simulink model "METI_CVT_Thermal_ver01_2015a"  (R2015a)
settings: Solver=ode8  SolverMode=SingleTasking  StartTime=0  StopTime=1204  FixedStep=sampling_time  RelTol=1e-3
PreLoadFcn:
  | init_setting;
values from neighbouring files (symbols this model uses):
  degC2K = 273.15    [METI_TRAMI_Thermal_ver01_Jmaab_PreLoad.m]    (also in init_setting_METI.m)
  K2degC = -273.15    [METI_TRAMI_Thermal_ver01_Jmaab_PreLoad.m]    (also in init_setting_METI.m)
  sampling_time = 0.0025    [METI_TRAMI_Thermal_ver01_Jmaab_PreLoad.m]
undefined symbols (not defined in the file or in its folder): ALT_CNT_ALT_OFF_RPM_HYS_rpm, ALT_CNT_ALT_ON_RPM_HYS_rpm, ALT_CNT_Alter_V_BASE_V, ALT_CNT_Alter_V_Kaisei_V, ALT_CNT_flag_disable_kaisei, ALT_CNT_V_Battely_Kudo_V, ALT_PNT_ALT_GDCurrent_A, ALT_PNT_ALT_GDVolt_V, ALT_PNT_Alter_limit_Current_V_table, ALT_PNT_Alter_limit_Current_V_table_x_rpm, ALT_PNT_Alter_trq_Nm_map, ALT_PNT_Alter_trq_Nm_map_x_rpm, ALT_PNT_Alter_trq_Nm_map_y_Current_A, ALT_PNT_Alter_trq_Nm_map_z_Volt_tgt_V, ALT_PNT_eta_pulley_alt, ALT_PNT_Gain_Alt_v_del, ALT_PNT_ratio_pulley_alt, ALT_PNT_Tau_Alternator_V_tgt_s, ALT_PNT_trq_alter_output_LL_Nm, BK_PNT_Pow_UL, BK_PNT_Tau_brake, Brk_LL, Brk_PGain, Brk_UL, BT_PNT_Lo_Capa_lo_batt_F, BT_PNT_Lo_ocv_SOC_lo_batt_OCV_V_table, BT_PNT_Lo_ocv_SOC_lo_batt_OCV_V_table_x_SOC, BT_PNT_Lo_R_lo_batt_ohm, BT_PNT_Lo_SOC_MAX_lo_batt, BT_PNT_Lo_SOC_MIN_lo_batt, BT_PNT_Lo_SOC_START_lo_batt, DF_PNT_DF_gear, DF_PNT_DFBlock2DFAir_Heat_Resi_KpW, DF_PNT_DFBlock_Heat_Capa_JpK, DF_PNT_DFBlock_Temp_ini_degC, DF_PNT_DFOil2DFBlock_Heat_Resi_KpW, DF_PNT_DFOil_Heat_Capa_JpK, DF_PNT_DFOil_Temp_ini_degC, DF_PNT_Driveshaft_damper, DF_PNT_Driveshaft_delta_radps_LL, DF_PNT_Driveshaft_delta_radps_UL, DF_PNT_Driveshaft_spring, DF_PNT_eta_DF, DF_PNT_Outtemp_degC, DF_PNT_TMBlock2DFBlock_Heat_Resi_KpW, Driver_Brake_Const1, Driver_Brake_Const3, Driver_Brake_Switch_Const2, Driver_Brk_sh, drivmode_ACC, drivmode_CONST, drivmode_GensokuKaisei, drivmode_GensokuRikko, drivmode_STOP, EL_PNT_R_bodyelec_lo_ohm, ENG_CNT_acc_idlestop, ENG_CNT_Accel_LL, ENG_CNT_Accel_UL, ENG_CNT_brak_idlestop, ENG_CNT_flag_idle_stop_exe ... (+133)
undefined symbols (not defined in the file): ACC_D_Gain, ACC_I_Gain, ACC_P_Gain
libraries: METI_Lib_vehicle_model x32, simulink x7, AZAPA_Lib_vehicle_model x1
(part 1 of 3)
settings Model: CovSFcnEnable=off  Creator=nishimura  LastModifiedBy=AZ064
settings OptimizationCC: BlockReduction=off  BooleanDataType=off  EfficientMapNaN2IntZero=off
settings DebuggingCC: SaveWithParameterizedLinksMsg=none  UnderspecifiedInitializationDetection=Classic  MergeDetectMultiDrivingBlocksExec=none  SignalResolutionControl=TryResolveAllWithWarning  StrictBusMsg=ErrorOnBusTreatedAsVector
settings HardwareCC: TargetLongLongMode=on  TargetIntDivRoundTo=Zero  TargetEndianess=LittleEndian  TargetHWDeviceType=MATLAB Host  ProdEqTarget=off
settings CodeAppCC: MaxIdLength=128
settings GRTTargetCC: CombineOutputUpdateFcns=off  GRTInterface=on

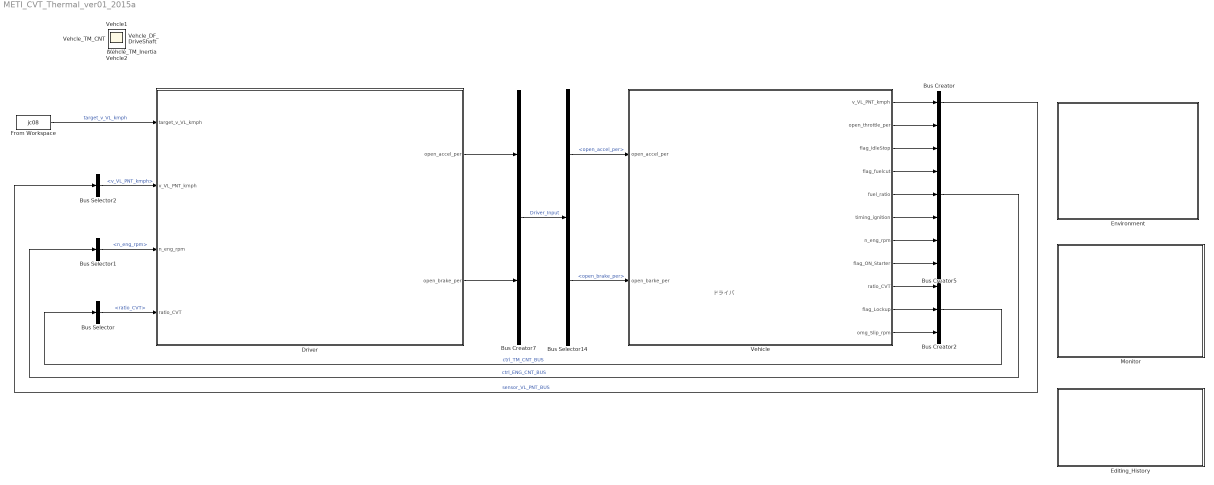
== system METI_CVT_Thermal_ver01_2015a ==
  note: ドライバ
  Bus Creator : BusCreator  Inputs=1
  Bus Creator2 : BusCreator  Inputs=3
  Bus Creator5 : BusCreator  Inputs=7
  Bus Creator7 : BusCreator  Inputs=2
  Bus Selector : BusSelector  OutputSignals=ratio_CVT
  Bus Selector1 : BusSelector  OutputSignals=n_eng_rpm
  Bus Selector14 : BusSelector  OutputSignals=open_accel_per,open_brake_per
  Bus Selector2 : BusSelector  OutputSignals=v_VL_PNT_kmph
  Driver : Subsystem
      mask Display: image(imread('picture\ドライバ.png'))
  Editing_History : Subsystem
  Environment : Subsystem
      mask Display: image(imread('picture\外部環境.png'))
  From Workspace : FromWorkspace  VariableName=jc08  SampleTime=0  OutputAfterFinalValue=Holding final value
  Monitor : Subsystem
  Vehicle : Subsystem
      mask Display: image(imread('picture\電気負荷.png'))
  Driver1 : Scope
      settings: YMin=-12.5  YMax=112.5  SaveName=ScopeData2
  Vehcle1 : Scope
      settings: YMin=-10  YMax=10  SaveName=ScopeData8
  Vehcle2 : Scope
      settings: YMin=-19.56201  YMax=196.87604
  Vehcle_DF_DriveShaft : Scope
      settings: YMin=-11.28415  YMax=101.55731  SaveName=ScopeData6
  Vehcle_TM_CNT : Scope
      settings: YMin=-0.125  YMax=1.125  SaveName=ScopeData8
  Vehcle_TM_Inertia : Scope
      settings: YMin=-138.01223  YMax=25.56889  SaveName=ScopeData7
  wires:
  From Workspace/1 -> Driver/1(target_v_VL_kmph)  "target_v_VL_kmph"
  Bus Creator7/1 -> Bus Selector14/1  "Driver_Input"
  Bus Creator/1 -> Bus Selector2/1  "sensor_VL_PNT_BUS"
  Bus Creator2/1 -> Bus Selector/1  "ctrl_TM_CNT_BUS"
  Bus Creator5/1 -> Bus Selector1/1  "ctrl_ENG_CNT_BUS"
  Vehicle/1(v_VL_PNT_kmph) -> Bus Creator/1
  Vehicle/2(open_throttle_per) -> Bus Creator5/1
  Vehicle/3(flag_IdleStop) -> Bus Creator5/2
  Vehicle/4(flag_fuelcut) -> Bus Creator5/3
  Vehicle/5(fuel_ratio) -> Bus Creator5/4
  Vehicle/6(timing_ignition) -> Bus Creator5/5
  Vehicle/7(n_eng_rpm) -> Bus Creator5/6
  Vehicle/8(flag_ON_Starter) -> Bus Creator5/7
  Vehicle/10(flag_Lockup) -> Bus Creator2/2
  Vehicle/9(ratio_CVT) -> Bus Creator2/1
  Vehicle/11(omg_Slip_rpm) -> Bus Creator2/3
  Bus Selector14/1 -> Vehicle/1(open_accel_per)  "<open_accel_per>"
  Bus Selector14/2 -> Vehicle/2(open_barke_per)  "<open_brake_per>"
  Driver/1(open_accel_per) -> Bus Creator7/1
  Driver/2(open_brake_per) -> Bus Creator7/2
  Bus Selector/1 -> Driver/4(ratio_CVT)  "<ratio_CVT>"
  Bus Selector1/1 -> Driver/3(n_eng_rpm)  "<n_eng_rpm>"
  Bus Selector2/1 -> Driver/2(v_VL_PNT_kmph)  "<v_VL_PNT_kmph>"

== system METI_CVT_Thermal_ver01_2015a/Driver ==
  note: ドライバモデルのへたくそ対応
  note: 全体としてパワーを算出しておいて、
      | さらにパワーと速度のF/Bを切り替えれるようにしておく
  target_v_VL_kmph : Inport
  v_VL_PNT_kmph : Inport  Port=2
  n_eng_rpm : Inport  Port=3
  ratio_CVT : Inport  Port=4
  Caliculate_Driving_State : Subsystem
  Caliculate_Opeining_Accel : Subsystem
  Caliculate_Opening_Brake : Subsystem
  Memory2 : Memory  InheritSampleTime=on
  Memory3 : Memory
  Memory4 : Memory
  open_accel_per : Outport
  open_brake_per : Outport  Port=2
  tag scope: tScope_accel=global, tScope_brake=global
  wires:
  target_v_VL_kmph/1 -> Caliculate_Opeining_Accel/2(target_v_VL_kmph), Caliculate_Opening_Brake/2(target_v_VL_kmph), Caliculate_Driving_State/2(target_v_VL_kmph)
  Memory3/1 -> Caliculate_Opeining_Accel/3(pre_n_eng_rpm)  "pre_n_eng_rpm"
  ratio_CVT/1 -> Memory4/1
  Memory4/1 -> Caliculate_Opeining_Accel/4(pre_ratio_CVT)  "pre_ratio_CVT"
  n_eng_rpm/1 -> Memory3/1
  Memory2/1 -> Caliculate_Opening_Brake/1(v_VL_PNT_kmph), Caliculate_Opeining_Accel/1(v_VL_PNT_kmph)
  Caliculate_Opeining_Accel/1(open_accel_per) -> Caliculate_Opening_Brake/3(open_accel_per), open_accel_per/1, [tScope_accel]
  Caliculate_Opening_Brake/1(open_brake_per) -> Caliculate_Driving_State/1(open_brake_per), open_brake_per/1, [tScope_brake]
  v_VL_PNT_kmph/1 -> Memory2/1

== system METI_CVT_Thermal_ver01_2015a/Editing_History ==
  note: 編集履歴
      |
      | 2019/3/29　初版
      |
      | 2019/7/3　ver.2
      | ・ENG_CNT内部と出力の結線名を修正
      | ・DFとPTTH間の熱のI/Fを追加修正
      | ・PTTH_PNT/RDTH_PNTの絵が同梱されていなかったため追加

== system METI_CVT_Thermal_ver01_2015a/Environment ==
  note: 登坂。風、温度、湿度・・・
  Clock : Clock
  To Workspace : ToWorkspace  VariableName=simtime  SampleTime=-1
      settings: Decimation=num_tws_mabiki
  wires:
  Clock/1 -> To Workspace/1

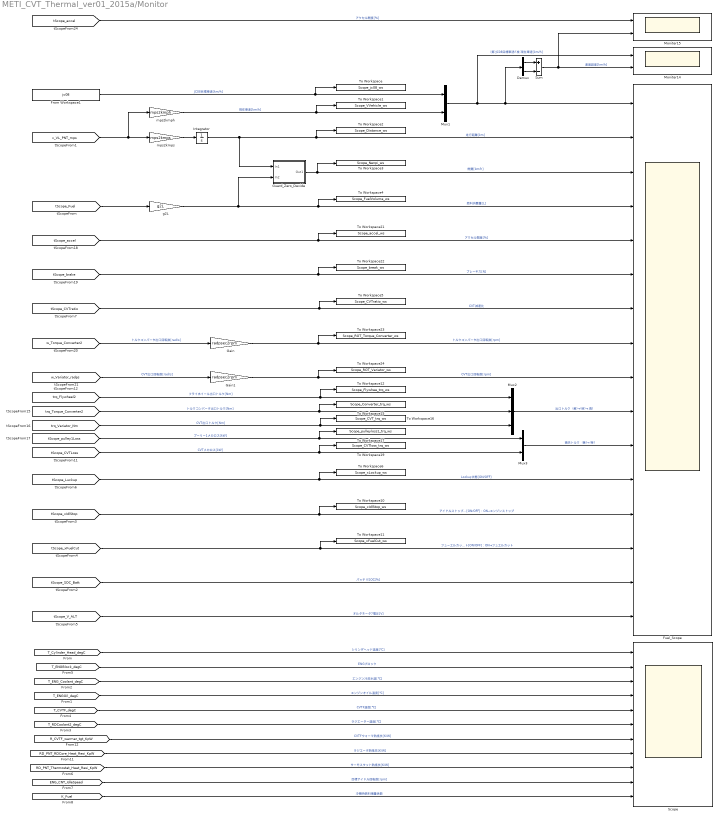
== system METI_CVT_Thermal_ver01_2015a/Monitor ==
  Demux : Demux  Outputs=2
  From Workspace1 : FromWorkspace  VariableName=jc08  SampleTime=0  OutputAfterFinalValue=Holding final value
  Fuel_Scope : Scope  NumInputPorts=16
      settings: YMin=0~0~0~0~0~0~0.25~0~0~-300~-500~0~0~0~99.6~9  YMax=75~5~20~0.3~20~100~2.5~4000~5000~300~3500~1~1~1~100.3~15
  Gain : Gain  Gain=radpsec2rpm
  Gain1 : Gain  Gain=radpsec2rpm
  Guard_Zero_Devide : Subsystem
  Integrator : Integrator
  Moniter14 : Scope  NumInputPorts=2
      settings: YMin=-10.20589~-3.34691  YMax=91.85305~1.30656
  Moniter15 : Scope  NumInputPorts=2
      settings: YMin=-1.14178~-3.31361  YMax=10.27601~1.05767
  Mux1 : Mux  Inputs=2
  Mux2 : Mux  Inputs=3
  Mux3 : Mux  Inputs=2
  Scope : Scope  NumInputPorts=11
      settings: YMin=0~25~25~25~25~25~-5~-5~-5~-5~-5  YMax=1050~125~100~100~100~100~5~5~5~5~5  SaveName=ScopeData3  Decimation=10
  Sum : Sum  Inputs=+-
  To Workspace : ToWorkspace  VariableName=Scope_jc08_ws  SaveFormat=Structure With Time  SampleTime=-1
      settings: Decimation=num_tws_mabiki
  To Workspace1 : ToWorkspace  VariableName=Scope_VVehicle_ws  SaveFormat=Structure With Time  SampleTime=-1
      settings: Decimation=num_tws_mabiki
  To Workspace10 : ToWorkspace  VariableName=Scope_xIdlStop_ws  SaveFormat=Structure With Time  SampleTime=-1
      settings: Decimation=num_tws_mabiki
  To Workspace11 : ToWorkspace  VariableName=Scope_xFuelCut_ws  SaveFormat=Structure With Time  SampleTime=-1
      settings: Decimation=num_tws_mabiki
  To Workspace12 : ToWorkspace  VariableName=Scope_Flywhee_trq_ws  SaveFormat=Structure With Time  SampleTime=-1
      settings: Decimation=num_tws_mabiki
  To Workspace15 : ToWorkspace  VariableName=Scope_Converter_trq_ws  SaveFormat=Structure With Time  SampleTime=-1
      settings: Decimation=num_tws_mabiki
  To Workspace16 : ToWorkspace  VariableName=Scope_CVT_trq_ws  SaveFormat=Structure With Time  SampleTime=-1
      settings: Decimation=num_tws_mabiki
  To Workspace17 : ToWorkspace  VariableName=Scope_pulleyloss1_trq_ws  SaveFormat=Structure With Time  SampleTime=-1
      settings: Decimation=num_tws_mabiki
  To Workspace19 : ToWorkspace  VariableName=Scope_CVTloss_trq_ws  SaveFormat=Structure With Time  SampleTime=-1
      settings: Decimation=num_tws_mabiki
  To Workspace2 : ToWorkspace  VariableName=Scope_Distance_ws  SaveFormat=Structure With Time  SampleTime=-1
      settings: Decimation=num_tws_mabiki
  To Workspace21 : ToWorkspace  VariableName=Scope_accel_ws  SaveFormat=Structure With Time  SampleTime=-1
      settings: Decimation=num_tws_mabiki
  To Workspace22 : ToWorkspace  VariableName=Scope_break_ws  SaveFormat=Structure With Time  SampleTime=-1
      settings: Decimation=num_tws_mabiki
  To Workspace23 : ToWorkspace  VariableName=Scope_ROT_Torque_Converter_ws  SaveFormat=Structure With Time  SampleTime=-1
      settings: Decimation=num_tws_mabiki
  To Workspace24 : ToWorkspace  VariableName=Scope_ROT_Variator_ws  SaveFormat=Structure With Time  SampleTime=-1
      settings: Decimation=num_tws_mabiki
  To Workspace3 : ToWorkspace  VariableName=Scope_Nenpi_ws  SaveFormat=Structure With Time  SampleTime=-1
      settings: Decimation=num_tws_mabiki
  To Workspace4 : ToWorkspace  VariableName=Scope_FuelVolume_ws  SaveFormat=Structure With Time  SampleTime=-1
      settings: Decimation=num_tws_mabiki
  To Workspace5 : ToWorkspace  VariableName=Scope_CVTratio_ws  SaveFormat=Structure With Time  SampleTime=-1
      settings: Decimation=num_tws_mabiki
  To Workspace6 : ToWorkspace  VariableName=Scope_xLockup_ws  SaveFormat=Structure With Time  SampleTime=-1
      settings: Decimation=num_tws_mabiki
  g2L : Gain  Gain=g2L
  mps2kmph : Gain  Gain=mps2kmph
  mps2kmps : Gain  Gain=mps2kmps
  wires:
  [tScope_xIdlStop] -> To Workspace10/1, Fuel_Scope/13  "アイドルストップ[ON/OFF] : ON→エンジンストップ"
  [tScope_xFuelCut] -> To Workspace11/1, Fuel_Scope/14  "フューエルカット[ON/OFF] : ON→フュエルカット"
  [v_VL_PNT_mps] -> mps2kmph/1, mps2kmps/1
  mps2kmps/1 -> Integrator/1
  [tScope_Fuel] -> g2L/1
  Integrator/1 -> Guard_Zero_Devide/1(In1), To Workspace2/1, Fuel_Scope/2  "走行距離[km]"
  g2L/1 -> To Workspace4/1, Fuel_Scope/4, Guard_Zero_Devide/2(In2)  "燃料消費量[L]"
  [tScope_Luckup] -> To Workspace6/1, Fuel_Scope/12  "Lockup状態[ON/OFF]"
  [tScope_CVTratio] -> To Workspace5/1, Fuel_Scope/7  "CVT減速比"
  From Workspace1/1 -> To Workspace/1, Mux1/1  "JC08目標車速[km/h]"
  mps2kmph/1 -> To Workspace1/1, Mux1/2  "現在車速[km/h]"
  Mux1/1 -> Moniter14/1, Demux/1, Fuel_Scope/1  "(黄)JC08目標車速/(桃)現在車速[km/h]"
  [tScope_CVTLoss] -> To Workspace19/1, Mux3/2  "CVTメカロス[kW]"
  [trq_Flywheel2] -> To Workspace12/1, Mux2/1  "フライホイール出口トルク[Nm]"
  [trq_Torque_Converter2] -> To Workspace15/1, Mux2/2  "トルクコンバータ出口トルク[Nm]"
  [trq_Variator_Nm] -> To Workspace16/1, Mux2/3  "CVT出口トルク[Nm]"
  [tScope_pulley1Loss] -> To Workspace17/1, Mux3/1  "プーリー1メカロス[kW]"
  Mux2/1 -> Fuel_Scope/10  "出口トルク  (黄)→(桃)→(青)"
  Mux3/1 -> Fuel_Scope/11  "損失トルク  (黄)→(桃)"
  [tScope_accel] -> To Workspace21/1, Fuel_Scope/5  "アクセル開度[%]"
  [tScope_brake] -> To Workspace22/1, Fuel_Scope/6  "ブレーキ力[N]"
  Gain/1 -> Fuel_Scope/8, To Workspace23/1  "トルクコンバータ出口回転数[rpm]"
  [w_Variator_radps] -> Gain1/1  "CVT出口回転数[rad/s]"
  Demux/1 -> Sum/1
  Demux/2 -> Sum/2
  Sum/1 -> Moniter14/2, Moniter15/2  "速度誤差[km/h]"
  [tScope_accel] -> Moniter15/1  "アクセル開度[%]"
  [tScope_V_ALT] -> Fuel_Scope/16  "オルタネータ7電圧[V]"
  [tScope_SOC_Batt] -> Fuel_Scope/15  "バッテリSOC[%]"
  Guard_Zero_Devide/1(Out1) -> To Workspace3/1, Fuel_Scope/3  "燃費[km/h]"
  [T_CVTF_degC] -> Scope/5  "CVTF温度[℃]"
  [T_RDCoolant2_degC] -> Scope/6  "ラジエーター温度[℃]"
  [T_ENG_Coolant_degC] -> Scope/3  "エンジン冷却水温[℃]"
  [T_ENGOil_degC] -> Scope/4  "エンジンオイル温度[℃]"
  [T_Cylinder_Head_degC] -> Scope/1  "シリンダヘッド温度[℃]"
  [T_ENGBlock_degC] -> Scope/2  "ENGブロック"
  [w_Torque_Converter2] -> Gain/1  "トルクコンバータ出口回転数[rad/s]"
  Gain1/1 -> To Workspace24/1, Fuel_Scope/9  "CVT出口回転数[rpm]"
  [R_CVTF_warmer_tgt_KpW] -> Scope/7  "CVTFウォーマ熱抵抗[K/W]"
  [RD_PNT_RDCore_Heat_Resi_KpW] -> Scope/8  "ラジエータ熱抵抗[K/W]"
  [RD_PNT_Thermostat_Heat_Resi_KpW] -> Scope/9  "サーモスタット熱抵抗[K/W]"
  [ENG_CNT_IdleSpeed] -> Scope/10  "目標アイドル回転数[rpm]"
  [K_Fuel] -> Scope/11  "冷機時燃料増量係数"

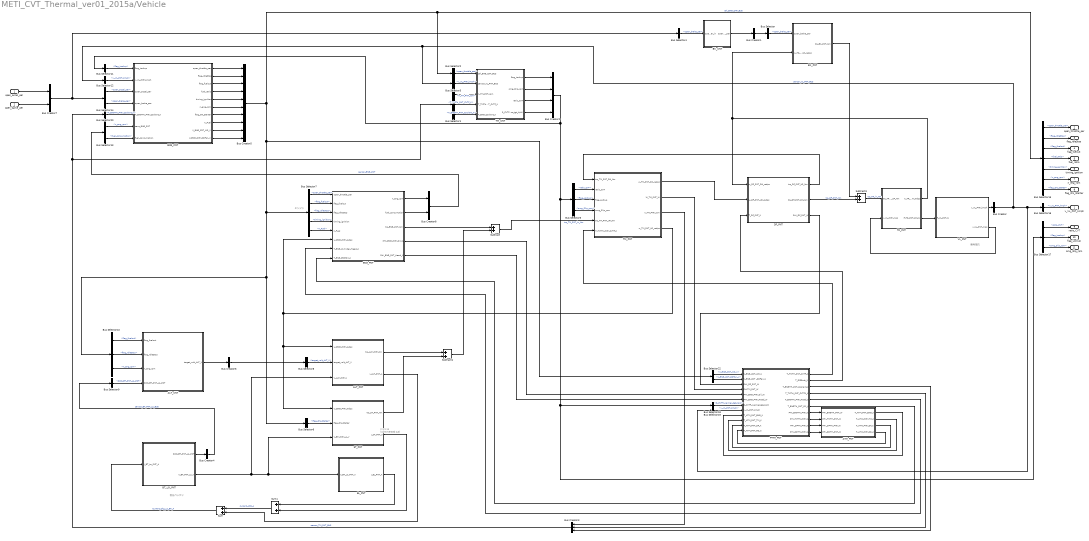
== system METI_CVT_Thermal_ver01_2015a/Vehicle ==
  note: エンジン
  note: 車両抵抗
  note: 低圧バッテリ
  open_accel_per : Inport
  open_barke_per : Inport  Port=2
  ALT_CNT : Subsystem
      mask Display: image(imread('picture\ECU.png'))
  ALT_PNT : Subsystem
      mask Display: image(imread('picture\image\オルタネータ02.jpg'))
  ATM_PNT : Subsystem
  BK_CNT : Subsystem
      mask Display: image(imread('picture\ECU.png'))
  BK_PNT : Subsystem
      mask Display: image(imread('picture\ブレーキ02.png'))
  BT_LO_PNT : Subsystem
      mask Display: image(imread('picture\バッテリー.png'))
  Bus Creator{,1,4,6} (4 alike) : BusCreator  Inputs=1
  Bus Creator2 : BusCreator
  Bus Creator3 : BusCreator  Inputs=3
  Bus Creator5 : BusCreator  Inputs=10
  Bus Creator7 : BusCreator  Inputs=2
  Bus Creator8 : BusCreator  Inputs=2
  Bus Selector : BusSelector  OutputSignals=open_brake_per
  Bus Selector1 : BusSelector  OutputSignals=n_TM_PNT_rpm,T_TMTH_PNT_CVTF_K,T_ENGTH_PNT_Coolant_K
  Bus Selector10 : BusSelector  OutputSignals=flag_fuelcut,flag_IdleStop,n_eng_rpm
  Bus Selector11 : BusSelector  OutputSignals=flag_Lockup
  Bus Selector{3,12,16,19} (4 alike) : BusSelector  OutputSignals=v_VL_PNT_kmph
  Bus Selector13 : BusSelector  OutputSignals=n_eng_rpm,fuel_consumption
  Bus Selector14 : BusSelector  OutputSignals=open_accel_per,open_brake_per
  Bus Selector15 : BusSelector  OutputSignals=open_throttle_per,flag_IdleStop,flag_fuelcut,fuel_ratio,timing_ignition,n_eng_rpm,flag_ON_Starter
  Bus Selector17 : BusSelector  OutputSignals=ratio_CVT,flag_Lockup,omg_Slip_rpm
  Bus Selector18 : BusSelector  OutputSignals=R_CVTF_warmer_tgt_KpW
  Bus Selector2 : BusSelector  OutputSignals=open_throttle_per
  Bus Selector20 : BusSelector  OutputSignals=T_ENGTH_PNT_Coolant_K
  Bus Selector22 : BusSelector  OutputSignals=V_ENG_CNT_WP_V,V_ENG_CNT_RDFan_V
  Bus Selector4 : BusSelector  OutputSignals=open_brake_per
  Bus Selector5 : BusSelector  OutputSignals=ratio_CVT,flag_Lockup,omg_Slip_rpm
  Bus Selector6 : BusSelector  OutputSignals=flag_ON_Starter
  Bus Selector7 : BusSelector  OutputSignals=open_throttle_per,flag_fuelcut,flag_IdleStop,timing_ignition,K_Fuel
  Bus Selector8 : BusSelector  OutputSignals=target_volt_ALT_V
  Bus Selector9 : BusSelector  OutputSignals=SOC_BT_PNT_Lo_PCT
  DF_PNT : Subsystem
      mask Display: image(imread('picture\回転変換.png'))
  EL_PNT : Subsystem
      mask Display: image(imread('picture\電気負荷.png'))
  ENG_CNT : Subsystem
      mask Display: image(imread('picture\ECU.png'))
  ENG_PNT : Subsystem
      mask Display: image(imread('picture\image\エンジン03.jpg'))
  From15 : From  Commented=on  GotoTag=I_ST_PNT_A  TagVisibility=global
  PTTH_PNT : Subsystem
  ST_PNT : Subsystem
      mask Display: image(imread('picture\image\スターター02.jpg'))
  Subtract : Sum  Inputs=2
  Subtract1 : Sum  Inputs=2
  Subtract3 : Sum  Inputs=2
  Sum : Sum
  Sum1 : Sum
  TM_CNT : Subsystem
      mask Display: image(imread('picture\ECU.png'))
  TM_PNT : Subsystem
      mask Display: image(imread('picture\image\トランスミッション02.jpg'))
  TR_PNT : Subsystem
      mask Display: image(imread('picture\タイヤ01.png'))
  VL_PNT : Subsystem
      mask Display: image(imread('picture\車両抵抗.png'))
  v_VL_PNT_kmph : Outport
  open_throttle_per : Outport  Port=2
  flag_IdleStop : Outport  Port=3
  flag_fuelcut : Outport  Port=4
  fuel_ratio : Outport  Port=5
  timing_ignition : Outport  Port=6
  n_eng_rpm : Outport  Port=7
  flag_ON_Starter : Outport  Port=8
  ratio_CVT : Outport  Port=9
  flag_Lockup : Outport  Port=10
  omg_Slip_rpm : Outport  Port=11
  wires:
  Bus Creator7/1 -> Bus Selector4/1, Bus Selector14/1
  Sum/1 -> BT_LO_PNT/1(I_BT_Lo_PNT_A)  "Current_Chg_Lo_BT_A"
  EL_PNT/1(I_EL_PNT_A) -> Sum1/1
  ALT_PNT/2(I_ALT_PNT_A) -> Sum/2
  Bus Creator5/1 -> Bus Selector15/1, Bus Selector2/1, Bus Selector22/1, Bus Selector7/1, Bus Selector6/1, Bus Selector10/1  "ctrl_ENG_CNT_BUS"
  Bus Creator6/1 -> Bus Selector8/1
  ST_PNT/2(I_ST_PNT_A) -> Sum1/2
  BT_LO_PNT/2(V_BT_PNT_Lo_V) -> ALT_PNT/3(V_ALT_PNT_V), EL_PNT/1(V_BT_Lo_PNT_V), ST_PNT/3(V_BT_PNT_Lo_V)
  Subtract/1 -> TM_PNT/5(trq_TM_PNT_UP_Nm)  "trq_TM_PNT_in_Nm"
  Bus Creator3/1 -> Bus Selector20/1, Bus Selector1/1  "sensor_TM_PNT_BUS"
  ENG_PNT/3(trq_ENG_PNT_Nm) -> Subtract/1
  Bus Creator2/1 -> Bus Selector17/1, Bus Selector18/1, Bus Selector5/1, Bus Selector11/1
  Bus Creator/1 -> Bus Selector16/1, Bus Selector19/1, Bus Selector3/1, Bus Selector12/1  "sensor_VL_PNT_BUS"
  BK_PNT/1(trq_BK_PNT_Nm) -> Subtract3/1
  TR_PNT/2(F_TR_PNT_DN_N) -> VL_PNT/1(F_VL_PNT_N)
  Subtract3/1 -> TR_PNT/1(trq_TR_PNT_UP_Nm)  "trq_TR_in_Nm"
  VL_PNT/2(v_VL_PNT_mps) -> TR_PNT/2(v_VL_PNT_mps)
  VL_PNT/1(v_VL_PNT_kmph) -> Bus Creator/1
  Bus Creator1/1 -> Bus Selector/1
  BK_CNT/1(open_brake_per) -> Bus Creator1/1
  Bus Selector/1 -> BK_PNT/1(open_brake_per)  "<open_brake_per>"
  Bus Selector1/1 -> TM_CNT/3(n_TM_PNT_rpm)  "<n_TM_PNT_rpm>"
  Bus Selector2/1 -> TM_CNT/1(ctrl_ENG_CNT_BUS)  "<open_throttle_per>"
  Bus Selector3/1 -> TM_CNT/2(sensor_VL_PNT_BUS)  "<v_VL_PNT_kmph>"
  TM_CNT/1(flag_Lockup) -> Bus Creator2/1
  TM_CNT/2(omg_Slip_rpm) -> Bus Creator2/2
  TM_CNT/3(ratio_CVT) -> Bus Creator2/3
  Bus Selector4/1 -> BK_CNT/1(open_brake_per_in)  "<open_brake_per>"
  Bus Selector5/1 -> TM_PNT/2(ratio_CVT)  "<ratio_CVT>"
  Bus Selector5/2 -> TM_PNT/3(flag_Lockup)  "<flag_Lockup>"
  Bus Selector5/3 -> TM_PNT/4(omg_Slip_rpm)  "<omg_Slip_rpm>"
  TM_PNT/3(n_TM_PNT_rpm) -> Bus Creator3/1
  Bus Creator4/1 -> Bus Selector9/1  "sensor_BT_PNT_Lo_BUS"
  BT_LO_PNT/1(SOC_BT_PNT_Lo_PCT) -> Bus Creator4/1
  Bus Selector6/1 -> ST_PNT/2(flag_ON_Starter)  "<flag_ON_Starter>"
  Bus Selector7/1 -> ENG_PNT/1(open_throttle_per)  "<open_throttle_per>"
  Bus Selector7/2 -> ENG_PNT/2(flag_fuelcut)  "<flag_fuelcut>"
  Bus Selector7/3 -> ENG_PNT/3(flag_IdleStop)  "<flag_IdleStop>"
  Bus Selector7/4 -> ENG_PNT/4(timing_ignition)  "<timing_ignition>"
  ENG_CNT/1(open_throttle_per) -> Bus Creator5/1
  ENG_CNT/7(flag_ON_Starter) -> Bus Creator5/7
  ENG_CNT/6(n_eng_rpm) -> Bus Creator5/6
  ENG_CNT/5(timing_ignition) -> Bus Creator5/5
  ENG_CNT/4(fuel_ratio) -> Bus Creator5/4
  ENG_CNT/3(flag_fuelcut) -> Bus Creator5/3
  ENG_CNT/2(flag_IdleStop) -> Bus Creator5/2
  Bus Selector8/1 -> ALT_PNT/2(target_volt_ALT_V)  "<target_volt_ALT_V>"
  ALT_CNT/1(target_volt_ALT_V) -> Bus Creator6/1
  Bus Selector9/1 -> ALT_CNT/4(SOC_BT_PNT_Lo_PCT)  "<SOC_BT_PNT_Lo_PCT>"
  Bus Selector10/1 -> ALT_CNT/1(flag_fuelcut)  "<flag_fuelcut>"
  Bus Selector10/2 -> ALT_CNT/2(flag_IdleStop)  "<flag_IdleStop>"
  Bus Selector10/3 -> ALT_CNT/3(n_eng_rpm)  "<n_eng_rpm>"
  Bus Selector11/1 -> ENG_CNT/1(flag_Lockup)  "<flag_Lockup>"
  Bus Selector12/1 -> ENG_CNT/2(v_VL_PNT_kmph)  "<v_VL_PNT_kmph>"
  Bus Selector13/1 -> ENG_CNT/6(sens_ENG_PNT)  "<n_eng_rpm>"
  Bus Selector14/1 -> ENG_CNT/3(open_accel_per)  "<open_accel_per>"
  Bus Selector14/2 -> ENG_CNT/4(open_brake_per)  "<open_brake_per>"
  Bus Selector16/1 -> v_VL_PNT_kmph/1  "<v_VL_PNT_kmph>"
  Bus Selector15/1 -> open_throttle_per/1  "<open_throttle_per>"
  Bus Selector15/3 -> flag_fuelcut/1  "<flag_fuelcut>"
  Bus Selector15/2 -> flag_IdleStop/1  "<flag_IdleStop>"
  Bus Selector15/4 -> fuel_ratio/1  "<fuel_ratio>"
  Bus Selector15/5 -> timing_ignition/1  "<timing_ignition>"
  Bus Selector15/6 -> n_eng_rpm/1  "<n_eng_rpm>"
  Bus Selector15/7 -> flag_ON_Starter/1  "<flag_ON_Starter>"
  Bus Selector17/1 -> ratio_CVT/1  "<ratio_CVT>"
  Bus Selector17/2 -> flag_Lockup/1  "<flag_Lockup>"
  Bus Selector17/3 -> omg_Slip_rpm/1  "<omg_Slip_rpm>"
  open_accel_per/1 -> Bus Creator7/1
  open_barke_per/1 -> Bus Creator7/2
  TM_PNT/4(w_TM_PNT_UP_radps) -> ALT_PNT/1(w_ENG_PNT_radps), ST_PNT/1(w_ENG_PNT_radps), ENG_PNT/6(w_ENG_PNT_radps)
  TM_PNT/1(w_TM_PNT_DN_radps) -> DF_PNT/2(w_DF_PNT_UP_radps)
  DF_PNT/1(trq_DF_PNT_UP_Nm) -> TM_PNT/1(trq_TM_PNT_DN_Nm)
  TR_PNT/1(w_TR_PNT_UP_radps) -> DF_PNT/1(w_DF_PNT_DN_radps), BK_PNT/2(w_TR_PNT_UP_radps)
  Sum1/1 -> Sum/1  "current_ACC_A"
  Subtract1/1 -> Subtract/2
  ST_PNT/1(trq_ST_PNT_Nm) -> Subtract1/2
  ALT_PNT/1(trq_ALT_PNT_Nm) -> Subtract1/1
  DF_PNT/3(PHI_DF_PNT_W) -> PTTH_PNT/3(PHI_DF_PNT_W)
  PTTH_PNT/4(T_TMTH_PNT_CVTF1_K) -> Bus Creator3/2
  Bus Selector1/2 -> TM_CNT/4(T_TMTH_PNT_CVTF_K)  "<T_TMTH_PNT_CVTF_K>"
  DF_PNT/2(trq_DF_PNT_DN_Nm) -> Subtract3/2  "trq_DF_PNT_Nm"
  Bus Selector18/1 -> PTTH_PNT/7(R_CVTF_warmer_tgt_KpW)  "<R_CVTF_warmer_tgt_KpW>"
  PTTH_PNT/1(T_TMTH_PNT_CVTF_K) -> TM_PNT/6(T_TMTH_PNT_CVTF_K)
  TM_PNT/2(W_TM_PNT_W) -> PTTH_PNT/4(PHITM_PNT_W)
  Bus Selector19/1 -> PTTH_PNT/8(v_VL_PNT_kmph)  "<v_VL_PNT_kmph>"
  PTTH_PNT/3(T_ENGTH_PNT_Coolant_K) -> Bus Creator3/3
  Bus Selector1/3 -> TM_CNT/5(T_ENG_Coolant_K)  "<T_ENGTH_PNT_Coolant_K>"
  Bus Selector20/1 -> ENG_CNT/5(T_ENGTH_PNT_Coolant_K)  "<T_ENGTH_PNT_Coolant_K>"
  ENG_CNT/8(K_Fuel) -> Bus Creator5/8
  Bus Selector7/5 -> ENG_PNT/5(K_Fuel)  "<K_Fuel>"
  Bus Selector13/2 -> ENG_CNT/7(fuel_consumption)  "<fuel_consumption>"
  ENG_PNT/4(PHI_ENG_PNT_Oil_W) -> PTTH_PNT/5(PHI_ENG_PNT_Oil_W)
  ENG_PNT/5(PHI_ENG_PNT_Head_W) -> PTTH_PNT/6(PHI_ENG_PNT_Head_W)
  PTTH_PNT/5(T_ENGTH_PNT_Head_K) -> ENG_PNT/7(T_ENG_Cylinder_Head_K)
  PTTH_PNT/6(T_ENGTH_PNT_Oil_K) -> ENG_PNT/8(T_ENG_ENGOil_K)
  ENG_CNT/9(V_ENG_CNT_WP_V) -> Bus Creator5/9
  Bus Selector22/2 -> PTTH_PNT/2(V_ENG_CNT _RDFan_V)  "<V_ENG_CNT_RDFan_V>"
  Bus Selector22/1 -> PTTH_PNT/1(V_ENG_CNT_WP_V)  "<V_ENG_CNT_WP_V>"
  Bus Creator8/1 -> Bus Selector13/1  "sensor_ENG_PNT"
  ENG_PNT/1(n_eng_rpm) -> Bus Creator8/1
  ENG_PNT/2(fuel_consumption) -> Bus Creator8/2
  PTTH_PNT/7(PHI_ENGTH_PNT_W) -> ATM_PNT/1(PHI_ENGTH_PNT_W)
  PTTH_PNT/8(PHI_TMTH_PNT_W) -> ATM_PNT/2(PHI_TMTH_PNT_W)
  PTTH_PNT/9(PHI_DFTH_PNT_W) -> ATM_PNT/3(PHI_DFTH_PNT_W)
  PTTH_PNT/10(PHI_RDTH_PNT_W) -> ATM_PNT/4(PHI_RDTH_PNT_W)
  ATM_PNT/1(T_ATM_PNT_ENG_K) -> PTTH_PNT/9(T_ATM_PNT_ENG_K)
  ATM_PNT/2(T_ATM_PNT_TM_K) -> PTTH_PNT/10(T_ATM_PNT_TM_K)
  ATM_PNT/3(T_ATM_PNT_DF_K) -> PTTH_PNT/11(T_ATM_PNT_DF_K)
  ATM_PNT/4(T_ATM_PNT_RD_K) -> PTTH_PNT/12(T_ATM_PNT_RD_K)
  TM_CNT/4(R_CVTF_warmer_tgt_KpW) -> Bus Creator2/4
  PTTH_PNT/2(T_DFBlock_K) -> DF_PNT/3(T_DF_PNT_K)
  ENG_CNT/10(V_ENG_CNT_RDFan_V) -> Bus Creator5/10

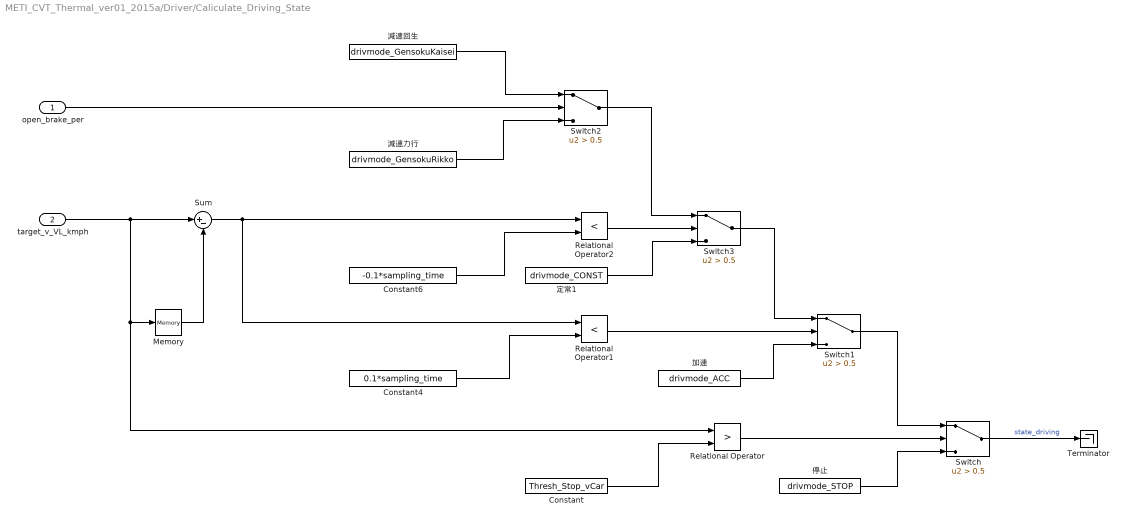
== system METI_CVT_Thermal_ver01_2015a/Driver/Caliculate_Driving_State ==
  open_brake_per : Inport
  target_v_VL_kmph : Inport  Port=2
  Constant : Constant  Value=Thresh_Stop_vCar
  Constant4 : Constant  Value=0.1*sampling_time
  Constant6 : Constant  Value=-0.1*sampling_time
  Memory : Memory
  Relational Operator : RelationalOperator  Operator=>  OutDataTypeStr=boolean
  Relational Operator1 : RelationalOperator  Operator=<  OutDataTypeStr=boolean
  Relational Operator2 : RelationalOperator  Operator=<  OutDataTypeStr=boolean
  Sum : Sum  Inputs=|+-
  Switch{,1..3} (4 alike) : Switch  Criteria=u2 > Threshold  Threshold=0.5
  Terminator : Terminator
  停止 : Constant  Value=drivmode_STOP
  加速 : Constant  Value=drivmode_ACC
  定常1 : Constant  Value=drivmode_CONST
  減速力行 : Constant  Value=drivmode_GensokuRikko
  減速回生 : Constant  Value=drivmode_GensokuKaisei
  wires:
  Switch/1 -> Terminator/1  "state_driving"
  target_v_VL_kmph/1 -> Relational Operator/1, Memory/1, Sum/1
  Relational Operator1/1 -> Switch1/2
  Constant4/1 -> Relational Operator1/2
  Relational Operator/1 -> Switch/2
  Constant/1 -> Relational Operator/2
  停止/1 -> Switch/3
  Sum/1 -> Relational Operator1/1, Relational Operator2/1
  減速回生/1 -> Switch2/1
  Switch3/1 -> Switch1/1
  Constant6/1 -> Relational Operator2/2
  Memory/1 -> Sum/2
  open_brake_per/1 -> Switch2/2
  減速力行/1 -> Switch2/3
  Relational Operator2/1 -> Switch3/2
  Switch2/1 -> Switch3/1
  定常1/1 -> Switch3/3
  加速/1 -> Switch1/3
  Switch1/1 -> Switch/1

== system METI_CVT_Thermal_ver01_2015a/Driver/Caliculate_Opeining_Accel ==
  v_VL_PNT_kmph : Inport
  target_v_VL_kmph : Inport  Port=2
  pre_n_eng_rpm : Inport  Port=3
  pre_ratio_CVT : Inport  Port=4
  FB : Subsystem  mask{P_Gain=ACC_P_Gain, D_Gain=ACC_D_Gain, I_Gain=ACC_I_Gain}
      mask prompts: P_Gain "Pゲイン値"; D_Gain "Dゲイン値"; I_Gain "Iゲイン値"
  FF : Subsystem
  Guard_0_100 : Saturate  UpperLimit=ENG_CNT_Throttle_UL  LowerLimit=ENG_CNT_Throttle_LL
  Sum1 : Sum  Inputs=|-+
  Sum3 : Sum  Inputs=++|
  open_accel_per : Outport
  wires:
  Sum1/1 -> FB/1(delta_v_VL_kmph)
  v_VL_PNT_kmph/1 -> FF/1(v_VL_PNT_kmph), Sum1/1
  target_v_VL_kmph/1 -> FF/2(target_v_VL_kmph), Sum1/2
  Sum3/1 -> Guard_0_100/1
  pre_n_eng_rpm/1 -> FF/3(pre_n_eng_rpm)
  pre_ratio_CVT/1 -> FF/4(pre_ratio_CVT)
  FB/1(FB_open_accel_per) -> Sum3/1
  FF/1(FF_open_accel_per) -> Sum3/2
  Guard_0_100/1 -> open_accel_per/1  "open_accel_per"

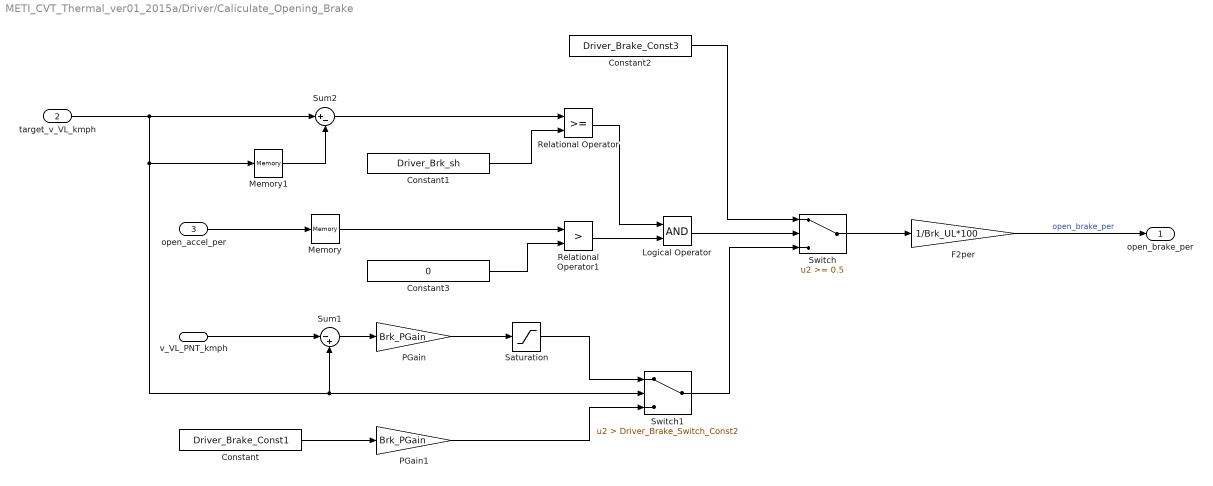
== system METI_CVT_Thermal_ver01_2015a/Driver/Caliculate_Opening_Brake ==
  v_VL_PNT_kmph : Inport
  target_v_VL_kmph : Inport  Port=2
  open_accel_per : Inport  Port=3
  Constant : Constant  Value=Driver_Brake_Const1
  Constant1 : Constant  Value=Driver_Brk_sh
  Constant2 : Constant  Value=Driver_Brake_Const3
  Constant3 : Constant  Value=0
  F2per : Gain  Gain=1/Brk_UL*100
  Logical Operator : Logic  AllPortsSameDT=off  OutDataTypeStr=boolean
  Memory : Memory
  Memory1 : Memory
  PGain : Gain  Gain=Brk_PGain
  PGain1 : Gain  Gain=Brk_PGain
  Relational Operator : RelationalOperator  OutDataTypeStr=boolean
  Relational Operator1 : RelationalOperator  Operator=>  OutDataTypeStr=boolean
  Saturation : Saturate  UpperLimit=Brk_UL  LowerLimit=Brk_LL
  Sum1 : Sum  Inputs=|-+
  Sum2 : Sum  Inputs=|+-
  Switch : Switch  Threshold=0.5
  Switch1 : Switch  Criteria=u2 > Threshold  Threshold=Driver_Brake_Switch_Const2
  open_brake_per : Outport
  wires:
  target_v_VL_kmph/1 -> Switch1/2, Sum1/2, Memory1/1, Sum2/1
  Sum1/1 -> PGain/1
  PGain/1 -> Saturation/1
  Constant/1 -> PGain1/1
  PGain1/1 -> Switch1/3
  open_accel_per/1 -> Memory/1
  Memory/1 -> Relational Operator1/1
  Memory1/1 -> Sum2/2
  Switch/1 -> F2per/1
  Sum2/1 -> Relational Operator/1
  Saturation/1 -> Switch1/1
  Switch1/1 -> Switch/3
  Constant2/1 -> Switch/1
  v_VL_PNT_kmph/1 -> Sum1/1
  Constant1/1 -> Relational Operator/2
  Constant3/1 -> Relational Operator1/2
  Relational Operator1/1 -> Logical Operator/2
  Relational Operator/1 -> Logical Operator/1
  Logical Operator/1 -> Switch/2
  F2per/1 -> open_brake_per/1  "open_brake_per"

== system METI_CVT_Thermal_ver01_2015a/Monitor/Guard_Zero_Devide ==
  note: 0割防止暫定処置
  In1 : Inport
  In2 : Inport  Port=2
  Constant1 : Constant  Value=fuel_0guard
  Constant2 : Constant  Value=fuelcomsnp_0
  Divide : Product  Inputs=*/
  MinMax : MinMax  Function=max  Inputs=2
  Relational Operator : RelationalOperator  OutDataTypeStr=boolean
  Switch1 : Switch  Criteria=u2 > Threshold  Threshold=0.5
  Out1 : Outport
  wires:
  In2/1 -> MinMax/1, Relational Operator/1
  In1/1 -> Divide/1
  Switch1/1 -> Out1/1  "燃費[km/l]"
  Divide/1 -> Switch1/1  "燃費[km/l]"
  Constant2/1 -> Switch1/3
  Relational Operator/1 -> Switch1/2
  MinMax/1 -> Divide/2
  Constant1/1 -> MinMax/2, Relational Operator/2

== system METI_CVT_Thermal_ver01_2015a/Vehicle/ALT_CNT ==
  note: 【発電禁止条件】
      | 下記条件いずれかが成立時はオルタネータの発電を禁止する
      |   (2)エンジン停止中
      |   (3)エンジン始動中(下記エンジン回転数で判定)
      |      ene ≦ ALT_ON_RPM_HYS(1000[rpm])
      |                    ヒスあり(400[rpm])
  note: 【強制回生モード切替条件】
  note: 【回生モード切替条件】
      | 減速時FC中
  note: 例) 12[V]
  note: 例) 14[V]
  note: 例) 13.5[V]
  flag_fuelcut : Inport
  flag_IdleStop : Inport  Port=2
  n_eng_rpm : Inport  Port=3
  SOC_BT_PNT_Lo_PCT : Inport  Port=4
  Constant : Constant  Value=ALT_CNT_Alter_V_Kaisei_V
  Constant1 : Constant  Value=ALT_CNT_V_Battely_Kudo_V
  Constant2 : Constant  Value=ALT_CNT_flag_disable_kaisei
  Constant3 : Constant  Value=ALT_CNT_Alter_V_BASE_V
  Constant4 : Constant  Value=BT_PNT_Lo_SOC_MAX_lo_batt
  Logical Operator : Logic  Operator=OR  Inputs=3  AllPortsSameDT=off  OutDataTypeStr=boolean
  Logical Operator1 : Logic  AllPortsSameDT=off  OutDataTypeStr=boolean
  Logical Operator2 : Logic  Operator=NOT  AllPortsSameDT=off  OutDataTypeStr=boolean
  Relational Operator : RelationalOperator  OutDataTypeStr=boolean
  Relay1 : Relay  OnSwitchValue=ALT_CNT_ALT_ON_RPM_HYS_rpm  OffSwitchValue=ALT_CNT_ALT_OFF_RPM_HYS_rpm  OnOutputValue=0  OffOutputValue=1
  Switch1 : Switch  Criteria=u2 > Threshold  Threshold=0.5
  Switch3 : Switch  Criteria=u2 > Threshold  Threshold=0.5
  target_volt_ALT_V : Outport
  wires:
  Constant1/1 -> Switch1/3
  Switch3/1 -> target_volt_ALT_V/1  "target_volt_ALT_V"
  Constant4/1 -> Relational Operator/2
  flag_IdleStop/1 -> Logical Operator/1
  Relay1/1 -> Logical Operator/2
  Relational Operator/1 -> Logical Operator/3
  Constant/1 -> Switch1/1
  flag_fuelcut/1 -> Logical Operator1/1
  Logical Operator/1 -> Logical Operator2/1
  Constant3/1 -> Switch3/1
  Constant2/1 -> Switch3/2
  Switch1/1 -> Switch3/3
  Logical Operator1/1 -> Switch1/2
  Logical Operator2/1 -> Logical Operator1/2
  n_eng_rpm/1 -> Relay1/1
  SOC_BT_PNT_Lo_PCT/1 -> Relational Operator/1

== system METI_CVT_Thermal_ver01_2015a/Vehicle/ALT_PNT ==
  note: 発電する為のトルクが負
  note: スルー量が出力の場合、発電する方向が正
  w_ENG_PNT_radps : Inport
  target_volt_ALT_V : Inport  Port=2
  V_ALT_PNT_V : Inport  Port=3
  Gain : Gain  Gain=-1
  Memory1 : Memory
  P_cal : METI_Lib_vehicle_model/P_cal  Type_energy=回転運動  Type_output_energy=出力  Power_name=Po_  t_Workspace_Name=ALT_PNT_MECK  P_VariableName=Po_ALT_PNT_MECK  Across_VariableName=w_ALT_PNT_MECK  Throgh_VariableName=tq_ALT_PNT_MECK
  P_cal1 : METI_Lib_vehicle_model/P_cal  Type_energy=電気  Type_output_energy=出力  Power_name=Po_  t_Workspace_Name=ALT_PNT_ELEC  P_VariableName=Po_ALT_PNT_ELEC  Across_VariableName=V_ALT_PNT_ELEC  Throgh_VariableName=I_ALT_PNT_ELEC
  Subsystem : Subsystem
  Terminator : Terminator
  Terminator1 : Terminator
  pulley_slave : Subsystem
  trq_ALT_PNT_Nm : Outport
  I_ALT_PNT_A : Outport  Port=2
  tag scope: tScope_V_ALT=global
  wires:
  Memory1/1 -> Subsystem/2(w_ROT_slavepulley12)
  Subsystem/1(current_ALT_PNT_A) -> P_cal1/2, I_ALT_PNT_A/1
  Gain/1 -> trq_ALT_PNT_Nm/1  "trq_ALT_PNT_Nm"
  pulley_slave/1(trq_slavepulley11) -> Gain/1
  w_ENG_PNT_radps/1 -> pulley_slave/1(w_ENG_PNT_radps)
  Subsystem/2(trq_trqsource) -> P_cal/2, pulley_slave/2(trq_slavepulley12)
  V_ALT_PNT_V/1 -> P_cal1/1, [tScope_V_ALT], Subsystem/3(volt_BT_PNT_Lo_V)
  P_cal1/1 -> Terminator1/1
  P_cal/1 -> Terminator/1
  pulley_slave/2(w_slavepulley12) -> P_cal/1, Memory1/1
  target_volt_ALT_V/1 -> Subsystem/1(target_volt_ALT_V)

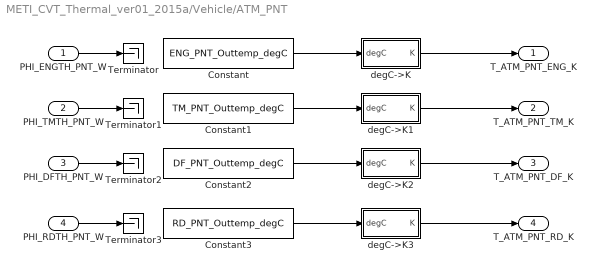
== system METI_CVT_Thermal_ver01_2015a/Vehicle/ATM_PNT ==
  PHI_ENGTH_PNT_W : Inport
  PHI_TMTH_PNT_W : Inport  Port=2
  PHI_DFTH_PNT_W : Inport  Port=3
  PHI_RDTH_PNT_W : Inport  Port=4
  Constant : Constant  Value=ENG_PNT_Outtemp_degC
  Constant1 : Constant  Value=TM_PNT_Outtemp_degC
  Constant2 : Constant  Value=DF_PNT_Outtemp_degC
  Constant3 : Constant  Value=RD_PNT_Outtemp_degC
  Terminator{,1..3} (4 alike) : Terminator
  degC->K : Subsystem
  degC->K1 : Subsystem
  degC->K2 : Subsystem
  degC->K3 : Subsystem
  T_ATM_PNT_ENG_K : Outport
  T_ATM_PNT_TM_K : Outport  Port=2
  T_ATM_PNT_DF_K : Outport  Port=3
  T_ATM_PNT_RD_K : Outport  Port=4
  wires:
  Constant/1 -> degC->K/1(degC)
  Constant1/1 -> degC->K1/1(degC)
  Constant2/1 -> degC->K2/1(degC)
  Constant3/1 -> degC->K3/1(degC)
  PHI_ENGTH_PNT_W/1 -> Terminator/1
  PHI_TMTH_PNT_W/1 -> Terminator1/1
  PHI_DFTH_PNT_W/1 -> Terminator2/1
  PHI_RDTH_PNT_W/1 -> Terminator3/1
  degC->K/1(K) -> T_ATM_PNT_ENG_K/1
  degC->K1/1(K) -> T_ATM_PNT_TM_K/1
  degC->K2/1(K) -> T_ATM_PNT_DF_K/1
  degC->K3/1(K) -> T_ATM_PNT_RD_K/1

== system METI_CVT_Thermal_ver01_2015a/Vehicle/BK_CNT ==
  open_brake_per_in : Inport
  open_brake_per : Outport
  wires:
  open_brake_per_in/1 -> open_brake_per/1

== system METI_CVT_Thermal_ver01_2015a/Vehicle/BK_PNT ==
  note: 制動力
  open_brake_per : Inport
  w_TR_PNT_UP_radps : Inport  Port=2
  Constant2 : Constant  Value=tire_r
  Gain : Gain  Gain=-1
  Product6 : Product  RndMeth=Zero
  Q_cal3 : METI_Lib_vehicle_model/P_cal  Type_energy=回転運動  Type_output_energy=損失  Power_name=Pl_  t_Workspace_Name=BK_PNT_MECK_LOSS  P_VariableName=Pl_BK_PNT_MECK_LOSS  Across_VariableName=w_BK_PNT_MECK_LOSS  Throgh_VariableName=tq_BK_PNT_MECK_LOSS
  Terminator1 : Terminator
  Transfer Fcn : TransferFcn  Denominator=[BK_PNT_Tau_brake 1]
  per2F : Gain  Gain=BK_PNT_Pow_UL/100
  trq_BK_PNT_Nm : Outport
  wires:
  Q_cal3/1 -> Terminator1/1
  Transfer Fcn/1 -> Product6/2
  Constant2/1 -> Product6/1
  Product6/1 -> Gain/1, Q_cal3/2
  w_TR_PNT_UP_radps/1 -> Q_cal3/1
  open_brake_per/1 -> per2F/1
  Gain/1 -> trq_BK_PNT_Nm/1  "trq_BK_PNT_Nm"
  per2F/1 -> Transfer Fcn/1

== system METI_CVT_Thermal_ver01_2015a/Vehicle/BT_LO_PNT ==
  note: SOC算出
  note: 内部抵抗
  note: OCV電圧算出
  I_BT_Lo_PNT_A : Inport
  Cal_SOC : Subsystem
  Capa_batt(Ah) : Constant  Value=BT_PNT_Lo_Capa_lo_batt_F
  Memory6 : Memory  InheritSampleTime=on
  P_cal : METI_Lib_vehicle_model/P_cal  Type_energy=電気  Type_output_energy=出力  Power_name=Po_  t_Workspace_Name=BT_PNT_Lo_ELEC  P_VariableName=Po_BT_PNT_Lo_ELEC  Across_VariableName=V_BT_PNT_Lo_ELEC  Throgh_VariableName=I_BT_PNT_Lo_ELEC
  P_cal1 : METI_Lib_vehicle_model/P_cal  Type_energy=電気  Type_output_energy=損失  Power_name=Pl_  t_Workspace_Name=BT_PNT_Lo_ELEC_LOSS  P_VariableName=Pl_BT_PNT_Lo_ELEC_LOSS  Across_VariableName=V_BT_PNT_Lo_ELEC_LOSS  Throgh_VariableName=I_BT_PNT_Lo_ELEC_LOSS
  SOC_MAX(%) : Constant  Value=BT_PNT_Lo_SOC_MAX_lo_batt
  SOC_MIN(%) : Constant  Value=BT_PNT_Lo_SOC_MIN_lo_batt
  SOC_START(%) : Constant  Value=BT_PNT_Lo_SOC_START_lo_batt
  Subsystem : Subsystem
  Sum : Sum
  Terminator1 : Terminator
  Terminator2 : Terminator
  map_OCV : Lookup  InputValues=BT_PNT_Lo_ocv_SOC_lo_batt_OCV_V_table_x_SOC  Table=BT_PNT_Lo_ocv_SOC_lo_batt_OCV_V_table  LookUpMeth=Interpolation-Use End Values
  SOC_BT_PNT_Lo_PCT : Outport
  V_BT_PNT_Lo_V : Outport  Port=2
  tag scope: tScope_SOC_Batt=global
  wires:
  Capa_batt(Ah)/1 -> Cal_SOC/2(Capa_batt)
  SOC_START(%)/1 -> Cal_SOC/3(SOC_st)
  SOC_MAX(%)/1 -> Cal_SOC/4(SOC_MAX)
  SOC_MIN(%)/1 -> Cal_SOC/5(SOC_MIN)
  Sum/1 -> V_BT_PNT_Lo_V/1, P_cal/1  "volt_BT_PNT_Lo_V"
  map_OCV/1 -> Sum/1
  Subsystem/1(V_BT_PNT_Lo_V) -> P_cal1/1, Sum/2
  P_cal/1 -> Terminator2/1
  P_cal1/1 -> Terminator1/1
  I_BT_Lo_PNT_A/1 -> Memory6/1, P_cal/2
  Cal_SOC/1(SOC_out) -> SOC_BT_PNT_Lo_PCT/1, map_OCV/1, [tScope_SOC_Batt]  "SOC_BT_PNT_Lo_PCT"
  Memory6/1 -> Subsystem/1(I_BT_PNT_Lo_A), P_cal1/2, Cal_SOC/1(I_Lo_BT_PNT_A)

== system METI_CVT_Thermal_ver01_2015a/Vehicle/DF_PNT ==
  note: DF効率
  note: 車両を動かす側が正
  w_DF_PNT_DN_radps : Inport
  w_DF_PNT_UP_radps : Inport  Port=2
  T_DF_PNT_K : Inport  Port=3
  Constant4 : Constant  Value=DF_PNT_DF_gear
  DriveShaft : Subsystem
  Product4 : Product  Inputs=*/  RndMeth=Zero
  Product7 : Product  Inputs=*/  RndMeth=Zero
  Q_cal1 : METI_Lib_vehicle_model/P_cal  Type_energy=回転運動  Type_output_energy=出力  Power_name=Po_  t_Workspace_Name=DF_PNT_MECK  P_VariableName=Po_DF_PNT_MECK  Across_VariableName=w_DF_PNT_MECK  Throgh_VariableName=tq_DF_PNT_MECK
  Q_cal4 : METI_Lib_vehicle_model/P_cal  Type_energy=回転運動  Type_output_energy=損失  Power_name=Pl_  t_Workspace_Name=DF_PNT_MECK_LOSS  P_VariableName=Pl_DF_PNT_MECK_LOSS  Across_VariableName=w_DF_PNT_MECK_LOSS  Throgh_VariableName=tq_DF_PNT_MECK_LOSS
  Terminator : Terminator
  Terminator3 : Terminator
  eta_DF : Constant  Value=DF_PNT_eta_DF
  eta_cal : METI_Lib_vehicle_model/eta_cal
  trq_DF_PNT_UP_Nm : Outport
  trq_DF_PNT_DN_Nm : Outport  Port=2
  PHI_DF_PNT_W : Outport  Port=3
  wires:
  w_DF_PNT_UP_radps/1 -> Product4/1, Q_cal4/1, Q_cal1/1
  eta_DF/1 -> eta_cal/1
  eta_cal/2 -> Q_cal1/2, trq_DF_PNT_UP_Nm/1  "trq_TM_PNT_Nm"
  eta_cal/1 -> Q_cal4/2
  Q_cal1/1 -> Terminator3/1
  Constant4/1 -> Product7/2, Product4/2
  Product7/1 -> eta_cal/2
  DriveShaft/1(trq_DS_PNT_in_Nm) -> trq_DF_PNT_DN_Nm/1
  Product4/1 -> DriveShaft/2(w_DS_PNT_in_radps)
  w_DF_PNT_DN_radps/1 -> DriveShaft/1(w_TR_PNT_radps)
  DriveShaft/2(trq_DF_PNT_Nm) -> Product7/1
  Q_cal4/1 -> PHI_DF_PNT_W/1
  T_DF_PNT_K/1 -> Terminator/1

== system METI_CVT_Thermal_ver01_2015a/Vehicle/EL_PNT ==
  note: 低圧側電気負荷
  V_BT_Lo_PNT_V : Inport
  Add : Sum  Inputs=+-
  Gain1 : Gain  Gain=-1
  Ground : Ground
  P_cal1 : METI_Lib_vehicle_model/P_cal  Type_energy=電気  Type_output_energy=損失  Power_name=Pl_  t_Workspace_Name=EL_PNT_ELEC_LOSS  P_VariableName=Pl_EL_PNT_ELEC_LOSS  Across_VariableName=V_EL_PNT_ELEC_LOSS  Throgh_VariableName=I_EL_PNT_ELEC_LOSS
  Product3 : Product  Inputs=*/  RndMeth=Zero
  Resistance2 : Constant  Value=EL_PNT_R_bodyelec_lo_ohm
  Terminator1 : Terminator
  I_EL_PNT_A : Outport
  wires:
  Product3/1 -> P_cal1/2, Gain1/1  "current_EL_PNT_A"
  V_BT_Lo_PNT_V/1 -> Add/1
  Ground/1 -> Add/2
  Add/1 -> Product3/1, P_cal1/1
  Resistance2/1 -> Product3/2
  P_cal1/1 -> Terminator1/1
  Gain1/1 -> I_EL_PNT_A/1

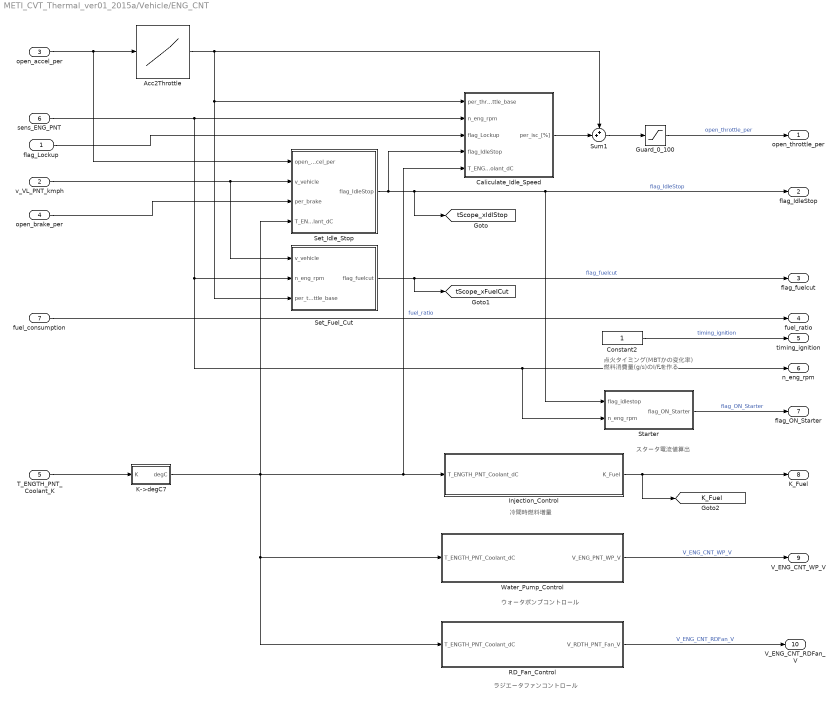
== system METI_CVT_Thermal_ver01_2015a/Vehicle/ENG_CNT ==
  note: 点火タイミング(MBTかの変化率)
      | 燃料消費量(g/s)のI/Fを作る
  note: スタータ電流値算出
  note: 冷間時燃料増量
  note: ウォータポンプコントロール
  note: ラジエータファンコントロール
  flag_Lockup : Inport
  v_VL_PNT_kmph : Inport  Port=2
  open_accel_per : Inport  Port=3
  open_brake_per : Inport  Port=4
  T_ENGTH_PNT_Coolant_K : Inport  Port=5
  sens_ENG_PNT : Inport  Port=6
  fuel_consumption : Inport  Port=7
  Acc2Throttle : Lookup_n-D  NumberOfTableDimensions=1  BreakpointsForDimension1=[ENG_CNT_Accel_LL:ENG_CNT_Accel_UL]  Table=[ENG_CNT_Throttle_LL:ENG_CNT_Throttle_UL]  RndMeth=Simplest  InputSameDT=on
  Caliculate_Idle_Speed : Subsystem
  Constant2 : Constant
  Guard_0_100 : Saturate  UpperLimit=ENG_CNT_Throttle_UL  LowerLimit=ENG_CNT_Throttle_LL
  Injection_Control : Subsystem
  K->degC7 : Subsystem
  RD_Fan_Control : Subsystem
  Set_Fuel_Cut : Subsystem
  Set_Idle_Stop : Subsystem
  Starter : Subsystem
  Sum1 : Sum  Inputs=++|
  Water_Pump_Control : Subsystem
  open_throttle_per : Outport
  flag_IdleStop : Outport  Port=2
  flag_fuelcut : Outport  Port=3
  fuel_ratio : Outport  Port=4
  timing_ignition : Outport  Port=5
  n_eng_rpm : Outport  Port=6
  flag_ON_Starter : Outport  Port=7
  K_Fuel : Outport  Port=8
  V_ENG_CNT_WP_V : Outport  Port=9
  V_ENG_CNT_RDFan_V : Outport  Port=10
  tag scope: K_Fuel=global, tScope_xFuelCut=global, tScope_xIdlStop=global
  wires:
  Set_Idle_Stop/1(flag_IdleStop) -> [tScope_xIdlStop], Starter/1(flag_idlestop), flag_IdleStop/1, Caliculate_Idle_Speed/4(flag_IdleStop)  "flag_IdleStop"
  Caliculate_Idle_Speed/1(per_isc_[%]) -> Sum1/2
  Sum1/1 -> Guard_0_100/1
  Acc2Throttle/1 -> Sum1/1, Caliculate_Idle_Speed/1(per_throttle_base), Set_Fuel_Cut/3(per_throttle_base)
  fuel_consumption/1 -> fuel_ratio/1  "fuel_ratio"
  Constant2/1 -> timing_ignition/1  "timing_ignition"
  Set_Fuel_Cut/1(flag_fuelcut) -> flag_fuelcut/1, [tScope_xFuelCut]  "flag_fuelcut"
  Guard_0_100/1 -> open_throttle_per/1  "open_throttle_per"
  sens_ENG_PNT/1 -> Caliculate_Idle_Speed/2(n_eng_rpm), Set_Fuel_Cut/2(n_eng_rpm), n_eng_rpm/1, Starter/2(n_eng_rpm)
  open_brake_per/1 -> Set_Idle_Stop/3(per_brake)
  open_accel_per/1 -> Acc2Throttle/1, Set_Idle_Stop/1(open_accel_per)
  v_VL_PNT_kmph/1 -> Set_Fuel_Cut/1(v_vehicle), Set_Idle_Stop/2(v_vehicle)
  Starter/1(flag_ON_Starter) -> flag_ON_Starter/1  "flag_ON_Starter"
  flag_Lockup/1 -> Caliculate_Idle_Speed/3(flag_Lockup)
  Water_Pump_Control/1(V_ENG_PNT_WP_V) -> V_ENG_CNT_WP_V/1  "V_ENG_CNT_WP_V"
  T_ENGTH_PNT_Coolant_K/1 -> K->degC7/1(K)
  Injection_Control/1(K_Fuel) -> [K_Fuel], K_Fuel/1
  RD_Fan_Control/1(V_RDTH_PNT_Fan_V) -> V_ENG_CNT_RDFan_V/1  "V_ENG_CNT_RDFan_V"
  K->degC7/1(degC) -> RD_Fan_Control/1(T_ENGTH_PNT_Coolant_dC), Water_Pump_Control/1(T_ENGTH_PNT_Coolant_dC), Set_Idle_Stop/4(T_ENGTH_PNT_Coolant_dC), Injection_Control/1(T_ENGTH_PNT_Coolant_dC), Caliculate_Idle_Speed/5(T_ENGTH_PNT_Coolant_dC)

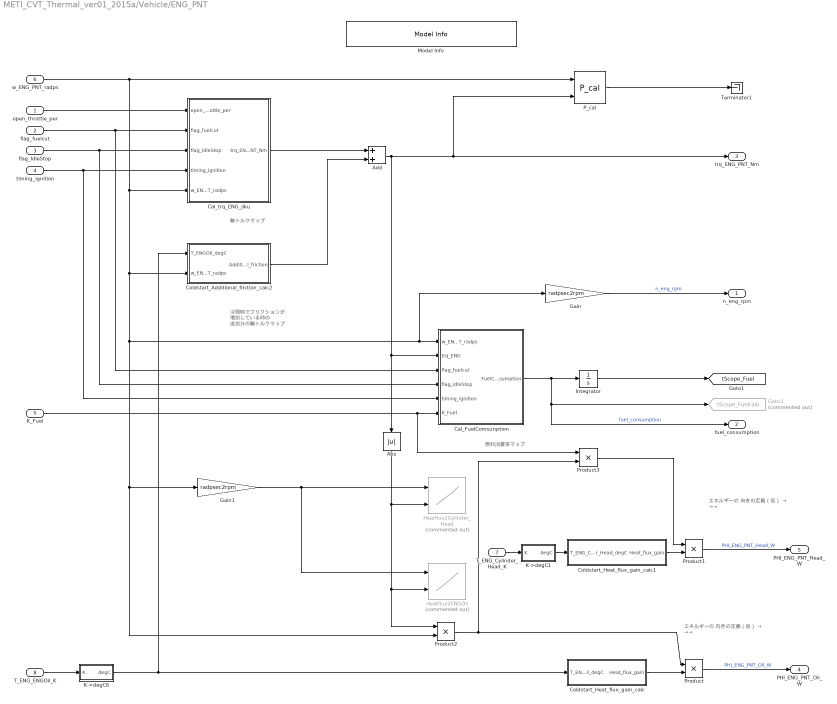
== system METI_CVT_Thermal_ver01_2015a/Vehicle/ENG_PNT ==
  note: 軸トルクマップ
  note: 燃料消費率マップ
  note: 冷間時でフリクションが
      | 増加している時の
      | 追加分の軸トルクマップ
  note: エネルギーの
      | 向きの定義（仮）
      | → →→
  note: エネルギーの
      | 向きの定義（仮）
      | → →→
  open_throttle_per : Inport
  flag_fuelcut : Inport  Port=2
  flag_IdleStop : Inport  Port=3
  timing_ignition : Inport  Port=4
  K_Fuel : Inport  Port=5
  w_ENG_PNT_radps : Inport  Port=6
  T_ENG_Cylinder_Head_K : Inport  Port=7
  T_ENG_ENGOil_K : Inport  Port=8
  Abs : Abs
  Add : Sum
  Cal_FuelComsunption : Subsystem
  Cal_trq_ENG_jiku : Subsystem
  Coldstart_Additional_friction_calc2 : Subsystem
  Coldstart_Heat_flux_gain_calc : Subsystem
  Coldstart_Heat_flux_gain_calc1 : Subsystem
  Gain : Gain  Gain=radpsec2rpm
  Gain1 : Gain  Gain=radpsec2rpm
  Goto3 : Goto  Commented=on  GotoTag=tScope_Fuelraio  TagVisibility=global
  Heatflux2Cylinder_Head : Lookup_n-D  Commented=on  BreakpointsForDimension1=ENG_PNT_Heatflux2Cylinder_Head_W_x_rpm  BreakpointsForDimension2=ENG_PNT_Heatflux2Cylinder_Head_W_y_trq  Table=ENG_PNT_Heatflux2Cylinder_Head_W  InternalRulePriority=Speed  RndMeth=Simplest  InputSameDT=on
  Heatflux2ENGOil : Lookup_n-D  Commented=on  BreakpointsForDimension1=ENG_PNT_Heatflux2ENGOil_W_x_rpm  BreakpointsForDimension2=ENG_PNT_Heatflux2ENGOil_W_y_trq  Table=ENG_PNT_Heatflux2ENGOil_W  InternalRulePriority=Speed  RndMeth=Simplest  InputSameDT=on
  Integrator : Integrator
  K->degC1 : Subsystem
  K->degC6 : Subsystem
  Model Info : simulink/Model-Wide Utilities/Model Info  Frame=on  DisplayStringWithTags=【注記】 ・エンジンモデルはトルク出力動作させる側が正  HorizontalTextAlignment=Left  LeftAlignmentValue=0.02  SourceBlockDiagram=METI_CVT_Thermal_ver01_2015a  TagMaxNumber=20
  P_cal : METI_Lib_vehicle_model/P_cal  Type_energy=回転運動  Type_output_energy=出力  Power_name=Po_  t_Workspace_Name=ENG_PNT_MECK  P_VariableName=Po_ENG_PNT_MECK  Across_VariableName=w_ENG_PNT_MECK  Throgh_VariableName=tq_ENG_PNT_MECK
  Product{,1..3} (4 alike) : Product
  Terminator1 : Terminator
  n_eng_rpm : Outport
  fuel_consumption : Outport  Port=2
  trq_ENG_PNT_Nm : Outport  Port=3
  PHI_ENG_PNT_Oil_W : Outport  Port=4
  PHI_ENG_PNT_Head_W : Outport  Port=5
  tag scope: tScope_Fuel=global
  wires:
  Cal_FuelComsunption/1(FuelConsumption) -> fuel_consumption/1, Goto3/1, Integrator/1  "fuel_consumption"
  Integrator/1 -> [tScope_Fuel]
  w_ENG_PNT_radps/1 -> P_cal/1, Coldstart_Additional_friction_calc2/2(w_ENG_PNT_radps), Gain1/1, Product2/2, Gain/1, Cal_FuelComsunption/1(w_ENG_PNT_radps), Cal_trq_ENG_jiku/5(w_ENG_PNT_radps)
  P_cal/1 -> Terminator1/1
  flag_fuelcut/1 -> Cal_trq_ENG_jiku/2(flag_fuelcut), Cal_FuelComsunption/3(flag_fuelcut)
  flag_IdleStop/1 -> Cal_FuelComsunption/4(flag_IdleStop), Cal_trq_ENG_jiku/3(flag_IdleStop)
  open_throttle_per/1 -> Cal_trq_ENG_jiku/1(open_throttle_per)
  Cal_trq_ENG_jiku/1(trq_ENG_PNT_Nm) -> Add/1
  timing_ignition/1 -> Cal_FuelComsunption/5(timing_ignition), Cal_trq_ENG_jiku/4(timing_ignition)
  Gain/1 -> n_eng_rpm/1  "n_eng_rpm"
  K->degC6/1(degC) -> Coldstart_Heat_flux_gain_calc/1(T_ENGOil_degC), Coldstart_Additional_friction_calc2/1(T_ENGOil_degC)
  T_ENG_Cylinder_Head_K/1 -> K->degC1/1(K)
  Product1/1 -> PHI_ENG_PNT_Head_W/1  "PHI_ENG_PNT_Head_W"
  Product/1 -> PHI_ENG_PNT_Oil_W/1  "PHI_ENG_PNT_Oil_W"
  Gain1/1 -> Heatflux2ENGOil/1, Heatflux2Cylinder_Head/1
  Coldstart_Heat_flux_gain_calc/1(Heat_flux_gain) -> Product/2
  Product2/1 -> Product/1, Product3/2
  Coldstart_Heat_flux_gain_calc1/1(Heat_flux_gain) -> Product1/2
  Coldstart_Additional_friction_calc2/1(Additional_friction) -> Add/2
  Add/1 -> trq_ENG_PNT_Nm/1, P_cal/2, Cal_FuelComsunption/2(trq_ENG), Abs/1
  K_Fuel/1 -> Product3/1, Cal_FuelComsunption/6(K_Fuel)
  Abs/1 -> Product2/1, Heatflux2ENGOil/2, Heatflux2Cylinder_Head/2
  Product3/1 -> Product1/1
  T_ENG_ENGOil_K/1 -> K->degC6/1(K)
  K->degC1/1(degC) -> Coldstart_Heat_flux_gain_calc1/1(T_ENG_Cylinder_Head_degC)

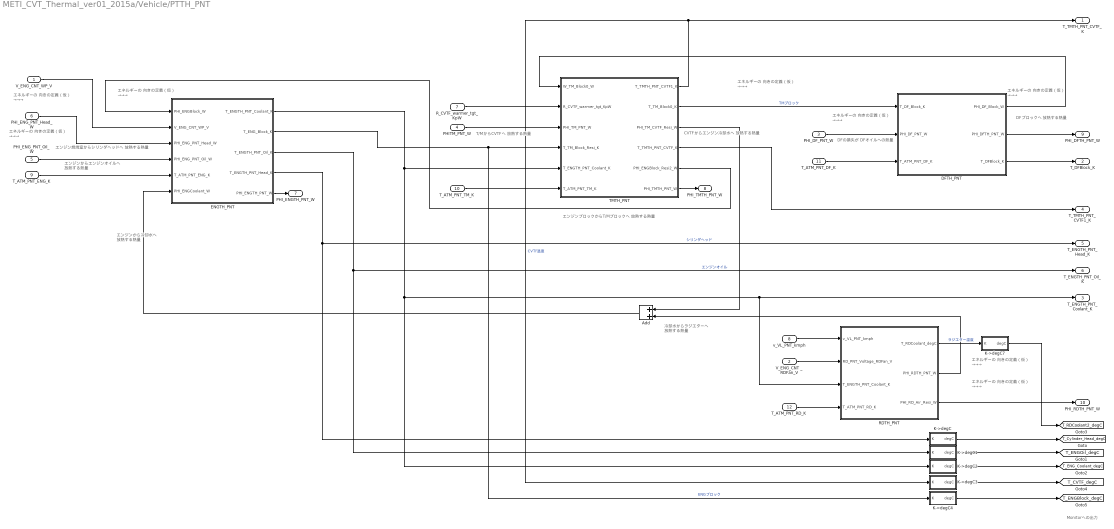
== system METI_CVT_Thermal_ver01_2015a/Vehicle/PTTH_PNT ==
  note: DFブロックへ
      | 放熱する熱量
  note: CVTFからエンジン冷却水へ
      | 放熱する熱量
  note: 冷却水からラジエターへ
      | 放熱する熱量
  note: エンジンブロックからT/Mブロックへ
      | 放熱する熱量
  note: エネルギーの
      | 向きの定義（仮）
      | →→→
  note: エネルギーの
      | 向きの定義（仮）
      | →→→
  note: エンジンから冷却水へ
      | 放熱する熱量
  note: エンジンからエンジンオイルへ
      | 放熱する熱量
  note: エネルギーの
      | 向きの定義（仮）
      | →→→
  note: エネルギーの
      | 向きの定義（仮）
      | →→→
  note: エネルギーの
      | 向きの定義（仮）
      | →→→
  note: エネルギーの
      | 向きの定義（仮）
      | →→→
  note: エネルギーの
      | 向きの定義（仮）
      | →→→
  note: エネルギーの
      | 向きの定義（仮）
      | →→→
  note: T/MからCVTFへ
      | 放熱する熱量
  note: Monitorへの出力
  note: DFの損失が
      | DFオイルへの熱量
  note: エンジン燃焼室からシリンダヘッドへ
      | 放熱する熱量
  V_ENG_CNT_WP_V : Inport
  V_ENG_CNT _RDFan_V : Inport  Port=2
  PHI_DF_PNT_W : Inport  Port=3
  PHITM_PNT_W : Inport  Port=4
  PHI_ENG_PNT_Oil_W : Inport  Port=5
  PHI_ENG_PNT_Head_W : Inport  Port=6
  R_CVTF_warmer_tgt_KpW : Inport  Port=7
  v_VL_PNT_kmph : Inport  Port=8
  T_ATM_PNT_ENG_K : Inport  Port=9
  T_ATM_PNT_TM_K : Inport  Port=10
  T_ATM_PNT_DF_K : Inport  Port=11
  T_ATM_PNT_RD_K : Inport  Port=12
  Add : Sum
  DFTH_PNT : Subsystem
      mask Display: image(imread('picture\回転変換.png'))
  ENGTH_PNT : Subsystem
      mask Display: image(imread('picture\image\エンジン03.jpg'))
  K->degC : Subsystem
  K->degC1 : Subsystem
  K->degC2 : Subsystem
  K->degC3 : Subsystem
  K->degC4 : Subsystem
  K->degC7 : Subsystem
  RDTH_PNT : Subsystem
      mask Display: image(imread('picture\ラジエーター_02s.jpg'))
  TMTH_PNT : Subsystem
      mask Display: image(imread('picture\image\トランスミッション02.jpg'))
  T_TMTH_PNT_CVTF_K : Outport
  T_DFBlock_K : Outport  Port=2
  T_ENGTH_PNT_Coolant_K : Outport  Port=3
  T_TMTH_PNT_CVTF1_K : Outport  Port=4
  T_ENGTH_PNT_Head_K : Outport  Port=5
  T_ENGTH_PNT_Oil_K : Outport  Port=6
  PHI_ENGTH_PNT_W : Outport  Port=7
  PHI_TMTH_PNT_W : Outport  Port=8
  PHI_DFTH_PNT_W : Outport  Port=9
  PHI_RDTH_PNT_W : Outport  Port=10
  tag scope: T_CVTF_degC=global, T_Cylinder_Head_degC=global, T_ENGBlock_degC=global, T_ENGOil_degC=global, T_ENG_Coolant_degC=global, T_RDCoolant2_degC=global
  wires:
  Add/1 -> ENGTH_PNT/6(PHI_ENGCoolant_W)
  RDTH_PNT/2(PHI_RDTH_PNT_W) -> Add/2
  TMTH_PNT/5(PHI_ENGBlock_Resi2_W) -> ENGTH_PNT/1(PHI_ENGBlock_W)
  ENGTH_PNT/2(T_ENG_Block_K) -> K->degC4/1(K), TMTH_PNT/4(T_TM_Block_Resi_K)  "ENGブロック"
  R_CVTF_warmer_tgt_KpW/1 -> TMTH_PNT/2(R_CVTF_warmer_tgt_KpW)
  ENGTH_PNT/4(T_ENGTH_PNT_Head_K) -> K->degC/1(K), T_ENGTH_PNT_Head_K/1  "シリンダヘッド"
  PHI_ENG_PNT_Head_W/1 -> ENGTH_PNT/3(PHI_ENG_PNT_Head_W)
  ENGTH_PNT/3(T_ENGTH_PNT_Oil_K) -> K->degC1/1(K), T_ENGTH_PNT_Oil_K/1  "エンジンオイル"
  PHI_ENG_PNT_Oil_W/1 -> ENGTH_PNT/4(PHI_ENG_PNT_Oil_W)
  PHITM_PNT_W/1 -> TMTH_PNT/3(PHI_TM_PNT_W)
  TMTH_PNT/1(T_TMTH_PNT_CVTF1_K) -> T_TMTH_PNT_CVTF_K/1, K->degC3/1(K)  "CVTF温度"
  TMTH_PNT/3(PHI_TM_CVTF_Resi_W) -> Add/1
  TMTH_PNT/2(T_TM_Block0_K) -> DFTH_PNT/1(T_DF_Block_K)  "TMブロック"
  v_VL_PNT_kmph/1 -> RDTH_PNT/1(v_VL_PNT_kmph)
  RDTH_PNT/1(T_RDCoolant_degC) -> K->degC7/1(K)  "ラジエター温度"
  V_ENG_CNT_WP_V/1 -> ENGTH_PNT/2(V_ENG_CNT_WP_V)
  V_ENG_CNT _RDFan_V/1 -> RDTH_PNT/2(RD_PNT_Voltage_RDFan_V)
  ENGTH_PNT/1(T_ENGTH_PNT_Coolant_K) -> K->degC2/1(K), T_ENGTH_PNT_Coolant_K/1, RDTH_PNT/3(T_ENGTH_PNT_Coolant_K), TMTH_PNT/5(T_ENGTH_PNT_Coolant_K)
  DFTH_PNT/1(PHI_DF_Block_W) -> TMTH_PNT/1(W_TM_Block0_W)
  PHI_DF_PNT_W/1 -> DFTH_PNT/2(PHI_DF_PNT_W)
  T_ATM_PNT_ENG_K/1 -> ENGTH_PNT/5(T_ATM_PNT_ENG_K)
  ENGTH_PNT/5(PHI_ENGTH_PNT_W) -> PHI_ENGTH_PNT_W/1
  TMTH_PNT/6(PHI_TMTH_PNT_W) -> PHI_TMTH_PNT_W/1
  T_ATM_PNT_TM_K/1 -> TMTH_PNT/6(T_ATM_PNT_TM_K)
  T_ATM_PNT_DF_K/1 -> DFTH_PNT/3(T_ATM_PNT_DF_K)
  DFTH_PNT/2(PHI_DFTH_PNT_W) -> PHI_DFTH_PNT_W/1
  T_ATM_PNT_RD_K/1 -> RDTH_PNT/4(T_ATM_PNT_RD_K)
  RDTH_PNT/3(PHI_RD_Air_Resi_W) -> PHI_RDTH_PNT_W/1
  TMTH_PNT/4(T_TMTH_PNT_CVTF_K) -> T_TMTH_PNT_CVTF1_K/1
  K->degC4/1(degC) -> [T_ENGBlock_degC]
  K->degC2/1(degC) -> [T_ENG_Coolant_degC]
  K->degC1/1(degC) -> [T_ENGOil_degC]
  K->degC/1(degC) -> [T_Cylinder_Head_degC]
  K->degC3/1(degC) -> [T_CVTF_degC]
  K->degC7/1(degC) -> [T_RDCoolant2_degC]
  DFTH_PNT/3(T_DFBlock_K) -> T_DFBlock_K/1

== system METI_CVT_Thermal_ver01_2015a/Vehicle/ST_PNT ==
  w_ENG_PNT_radps : Inport
  flag_ON_Starter : Inport  Port=2
  V_BT_PNT_Lo_V : Inport  Port=3
  Constant1 : Constant  Value=OFF
  Constant6 : Constant  Value=OFF
  Gain : Gain  Gain=1/ST_PNT_Starter_Res_ohm
  Gain1 : Gain  Gain=-1
  Switch : Switch  Criteria=u2 > Threshold  Threshold=0.5
  Terminator : Terminator
  trq_ST_PNT_Nm : Outport
  I_ST_PNT_A : Outport  Port=2
  wires:
  V_BT_PNT_Lo_V/1 -> Switch/1
  Switch/1 -> Gain/1
  Gain/1 -> Gain1/1  "current_ST_PNT_A"
  Constant6/1 -> Switch/3
  flag_ON_Starter/1 -> Switch/2
  Constant1/1 -> trq_ST_PNT_Nm/1  "trq__ST_PNT_Nm"
  w_ENG_PNT_radps/1 -> Terminator/1
  Gain1/1 -> I_ST_PNT_A/1
